simulink model "RobotDoSrodka10cmLimitZaokragloneNapSim"  (R2018a)
settings: Solver=ode45  StartTime=0.0  StopTime=tsym  RelTol=1e-6
values from neighbouring files (symbols this model uses):
  k1 = 10    [RobotDoSrodka10cmLimitZaokragloneNap.m]
  k2 = 100    [RobotDoSrodka10cmLimitZaokragloneNap.m]
  l = 0.0965    [RobotDoSrodka10cmLimitZaokragloneNap.m]
  R = 0.034    [RobotDoSrodka10cmLimitZaokragloneNap.m]
  wheelSpeedRadiansLimit = 8    [RobotDoSrodka10cmLimitZaokragloneNap.m]
undefined symbols (not defined in the file or in its folder): wd
settings Model: Creator=Papa Smerf  LastModifiedBy=Papa Smerf
settings DataIOCC: LimitDataPoints=on  SaveFormat=Array
settings OptimizationCC: BlockReduction=off  BooleanDataType=off  LifeSpan=inf
settings DebuggingCC: SaveWithParameterizedLinksMsg=none  UnderspecifiedInitializationDetection=Classic  MergeDetectMultiDrivingBlocksExec=none  SignalResolutionControl=TryResolveAllWithWarning  SFUnexpectedBacktrackingDiag=warning  SFNoUnconditionalDefaultTransitionDiag=warning  SFExecutionAtInitializationDiag=none
settings HardwareCC: ProdBitPerPointer=32  ProdBitPerSizeT=32  ProdBitPerPtrDiffT=32  ProdLargestAtomicFloat=None  ProdIntDivRoundTo=Undefined  ProdEndianess=Unspecified  ProdWordSize=32  ProdHWDeviceType=32-bit Generic  TargetUnknown=on
settings ModelReferenceCC: PropagateSignalLabelsOutOfModel=off
settings CodeAppCC: StateflowObjectComments=on
settings GRTTargetCC: TargetLangStandard=C89/C90 (ANSI)  GeneratePreprocessorConditionals=Disable all
settings ConfigComp: CovMetricSettings=dw  CovHtmlReporting=on  CovSaveCumulativeToWorkspaceVar=on  CovSaveSingleToWorkspaceVar=on  CovExternalEMLEnable=off  CovSFcnEnable=off

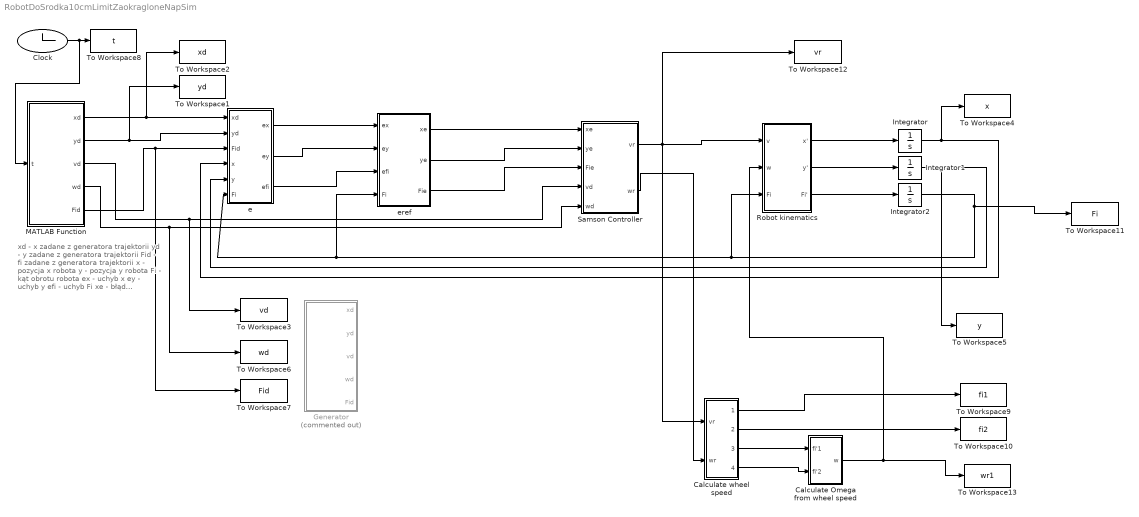
== system RobotDoSrodka10cmLimitZaokragloneNapSim ==
  note: xd - x zadane z generatora trajektorii
      | yd - y zadane z generatora trajektorii
      | Fid - fi zadane z generatora trajektorii
      | x - pozycja x robota
      | y - pozycja y robota
      | Fi - kąt obrotu robota
      | ex - uchyb x
      | ey - uchyb y
      | efi - uchyb Fi
      | xe - błąd referencyjny x
      | ye - błąd referencyjny y
      | Fie - błąd referencyjny Fi
      | vd - prędkość liniowa zadana
      | wd - prędkość kątowa zadana
      | vr - prędkość liniowa referencyjna
      | wr - prędkość kątowa referencyjna
      | v - prędkość liniowa zadana robota?
      | w - prędkość kątowa zadana robota?
      | x' - prędkość w osi x robota
      | y' - prędkość w osi y robota
      | Fi' - prędkość kątowa robota
  Calculate Omega from wheel speed : Subsystem
  Calculate wheel speed : Subsystem
  Clock : Clock
  Generator : Subsystem  Commented=on
  Integrator : Integrator
  Integrator1 : Integrator
  Integrator2 : Integrator
  MATLAB Function : MATLAB Function  TreatAsAtomicUnit=on
  Robot kinematics : Subsystem
  Samson Controller : Subsystem
  To Workspace1 : ToWorkspace  VariableName=yd  SampleTime=-1
  To Workspace10 : ToWorkspace  VariableName=fi2  SampleTime=0.01
  To Workspace11 : ToWorkspace  VariableName=Fi  SampleTime=0.01
  To Workspace12 : ToWorkspace  VariableName=vr  SampleTime=0.01
  To Workspace13 : ToWorkspace  VariableName=wr1  SampleTime=0.01
  To Workspace2 : ToWorkspace  VariableName=xd  SampleTime=-1
  To Workspace3 : ToWorkspace  VariableName=vd  SampleTime=-1
  To Workspace4 : ToWorkspace  VariableName=x  SampleTime=-1
  To Workspace5 : ToWorkspace  VariableName=y  SampleTime=-1
  To Workspace6 : ToWorkspace  VariableName=wd  SampleTime=-1
  To Workspace7 : ToWorkspace  VariableName=Fid  SampleTime=0.01
  To Workspace8 : ToWorkspace  VariableName=t  SampleTime=0.01
  To Workspace9 : ToWorkspace  VariableName=fi1  SampleTime=0.01
  e : Subsystem
  eref : Subsystem
  wires:
  e/1(ex) -> eref/1(ex)
  e/2(ey) -> eref/2(ey)
  e/3(efi) -> eref/3(efi)
  eref/1(xe) -> Samson Controller/1(xe)
  eref/2(ye) -> Samson Controller/2(ye)
  eref/3(Fie) -> Samson Controller/3(Fie)
  Robot kinematics/1(x') -> Integrator/1
  Robot kinematics/2(y') -> Integrator1/1
  Robot kinematics/3(Fi') -> Integrator2/1
  Integrator2/1 -> To Workspace11/1, Robot kinematics/3(Fi), e/6(Fi), eref/4(Fi)
  Integrator1/1 -> To Workspace5/1, e/5(y)
  Integrator/1 -> To Workspace4/1, e/4(x)
  MATLAB Function/1(xd) -> To Workspace2/1, e/1(xd)
  MATLAB Function/2(yd) -> To Workspace1/1, e/2(yd)
  MATLAB Function/5(Fid) -> To Workspace7/1, e/3(Fid)
  MATLAB Function/3(vd) -> To Workspace3/1, Samson Controller/4(vd)
  MATLAB Function/4(wd) -> To Workspace6/1, Samson Controller/5(wd)
  Clock/1 -> MATLAB Function/1(t), To Workspace8/1
  Calculate Omega from wheel speed/1(w) -> Robot kinematics/2(w), To Workspace13/1
  Calculate wheel speed/3(fi'1Rad) -> Calculate Omega from wheel speed/1(fi'1)
  Samson Controller/2(wr) -> Calculate wheel speed/2(wr)
  Calculate wheel speed/2(fi'2Obr) -> To Workspace10/1
  Calculate wheel speed/4(fi'2Rad) -> Calculate Omega from wheel speed/2(fi'2)
  Samson Controller/1(vr) -> Calculate wheel speed/1(vr), To Workspace12/1, Robot kinematics/1(v)
  Calculate wheel speed/1(fi'1Obr) -> To Workspace9/1

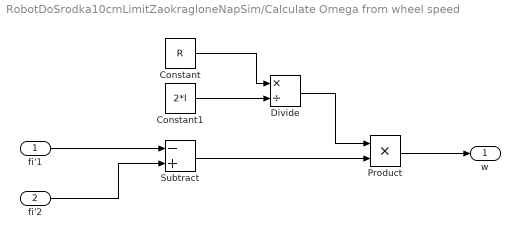
== system RobotDoSrodka10cmLimitZaokragloneNapSim/Calculate Omega from wheel speed ==
  fi'1 : Inport
  fi'2 : Inport  Port=2
  Constant : Constant  Value=R
  Constant1 : Constant  Value=2*l
  Divide : Product  Inputs=*/
  Product : Product
  Subtract : Sum  Inputs=-+
  w : Outport
  wires:
  Constant/1 -> Divide/1
  Product/1 -> w/1
  Subtract/1 -> Product/2
  Constant1/1 -> Divide/2
  fi'2/1 -> Subtract/2
  fi'1/1 -> Subtract/1
  Divide/1 -> Product/1

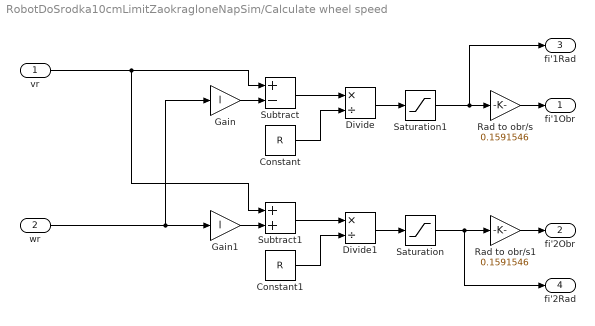
== system RobotDoSrodka10cmLimitZaokragloneNapSim/Calculate wheel speed ==
  vr : Inport
  wr : Inport  Port=2
  Constant : Constant  Value=R
  Constant1 : Constant  Value=R
  Divide : Product  Inputs=*/
  Divide1 : Product  Inputs=*/
  Gain : Gain  Gain=l
  Gain1 : Gain  Gain=l
  Rad to obr/s : Gain  Gain=0.1591546
  Rad to obr/s1 : Gain  Gain=0.1591546
  Saturation : Saturate  UpperLimit=wheelSpeedRadiansLimit  LowerLimit=-wheelSpeedRadiansLimit
  Saturation1 : Saturate  UpperLimit=wheelSpeedRadiansLimit  LowerLimit=-wheelSpeedRadiansLimit
  Subtract : Sum  Inputs=+-
  Subtract1 : Sum
  fi'1Obr : Outport
  fi'2Obr : Outport  Port=2
  fi'1Rad : Outport  Port=3
  fi'2Rad : Outport  Port=4
  wires:
  Rad to obr/s/1 -> fi'1Obr/1
  wr/1 -> Gain/1, Gain1/1
  Constant1/1 -> Divide1/2
  Subtract1/1 -> Divide1/1
  Gain/1 -> Subtract/2
  Constant/1 -> Divide/2
  Subtract/1 -> Divide/1
  Gain1/1 -> Subtract1/2
  Divide/1 -> Saturation1/1
  Divide1/1 -> Saturation/1
  Rad to obr/s1/1 -> fi'2Obr/1
  vr/1 -> Subtract1/1, Subtract/1
  Saturation/1 -> fi'2Rad/1, Rad to obr/s1/1
  Saturation1/1 -> fi'1Rad/1, Rad to obr/s/1

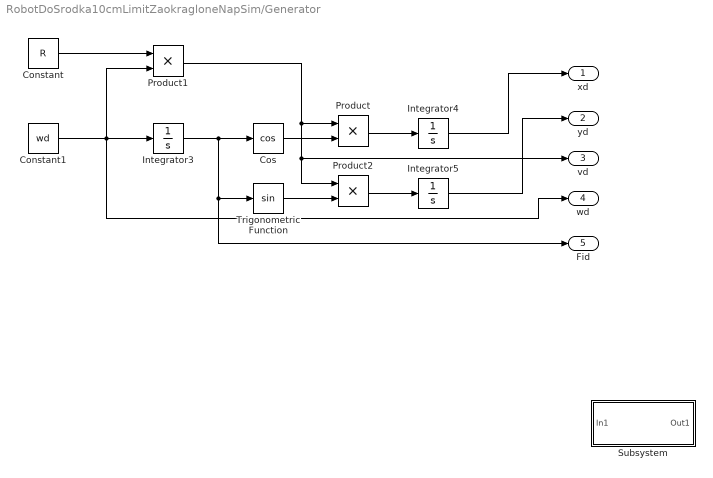
== system RobotDoSrodka10cmLimitZaokragloneNapSim/Generator ==
  Constant : Constant  Value=R
  Constant1 : Constant  Value=wd
  Cos : Trigonometry  Operator=cos
  Integrator3 : Integrator
  Integrator4 : Integrator
  Integrator5 : Integrator  InitialCondition=-R
  Product : Product
  Product1 : Product
  Product2 : Product
  Subsystem : Subsystem
  Trigonometric Function : Trigonometry
  xd : Outport
  yd : Outport  Port=2
  vd : Outport  Port=3
  wd : Outport  Port=4
  Fid : Outport  Port=5
  wires:
  Integrator5/1 -> yd/1
  Product1/1 -> vd/1, Product2/1, Product/1
  Constant/1 -> Product1/1
  Integrator3/1 -> Fid/1, Trigonometric Function/1, Cos/1
  Trigonometric Function/1 -> Product2/2
  Product/1 -> Integrator4/1
  Constant1/1 -> wd/1, Product1/2, Integrator3/1
  Cos/1 -> Product/2
  Integrator4/1 -> xd/1
  Product2/1 -> Integrator5/1

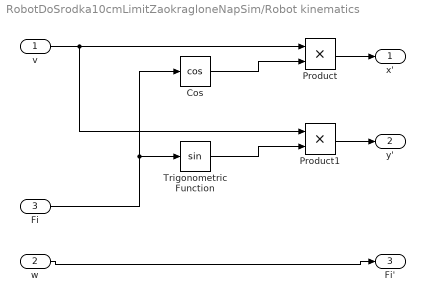
== system RobotDoSrodka10cmLimitZaokragloneNapSim/Robot kinematics ==
  v : Inport
  w : Inport  Port=2
  Fi : Inport  Port=3
  Cos : Trigonometry  Operator=cos
  Product : Product
  Product1 : Product
  Trigonometric Function : Trigonometry
  x' : Outport
  y' : Outport  Port=2
  Fi' : Outport  Port=3
  wires:
  w/1 -> Fi'/1
  Fi/1 -> Cos/1, Trigonometric Function/1
  Product1/1 -> y'/1
  v/1 -> Product1/1, Product/1
  Cos/1 -> Product/2
  Product/1 -> x'/1
  Trigonometric Function/1 -> Product1/2

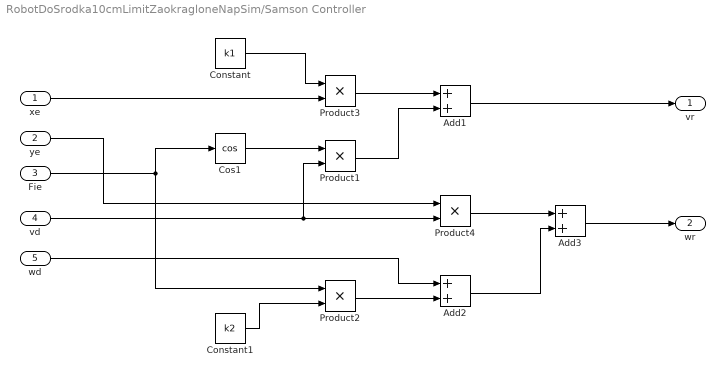
== system RobotDoSrodka10cmLimitZaokragloneNapSim/Samson Controller ==
  xe : Inport
  ye : Inport  Port=2
  Fie : Inport  Port=3
  vd : Inport  Port=4
  wd : Inport  Port=5
  Add1 : Sum
  Add2 : Sum
  Add3 : Sum
  Constant : Constant  Value=k1
  Constant1 : Constant  Value=k2
  Cos1 : Trigonometry  Operator=cos
  Product{1..4} (4 alike) : Product
  vr : Outport
  wr : Outport  Port=2
  wires:
  ye/1 -> Product4/1
  Fie/1 -> Product2/1, Cos1/1
  vd/1 -> Product4/2, Product1/2
  Add2/1 -> Add3/2
  Cos1/1 -> Product1/1
  xe/1 -> Product3/2
  Product3/1 -> Add1/1
  Product2/1 -> Add2/2
  Product1/1 -> Add1/2
  Add3/1 -> wr/1
  Add1/1 -> vr/1
  Constant/1 -> Product3/1
  Constant1/1 -> Product2/2
  wd/1 -> Add2/1
  Product4/1 -> Add3/1

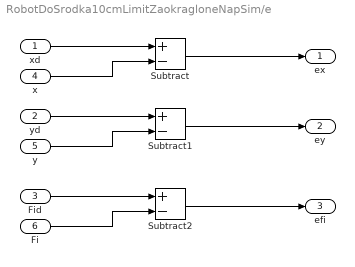
== system RobotDoSrodka10cmLimitZaokragloneNapSim/e ==
  xd : Inport
  yd : Inport  Port=2
  Fid : Inport  Port=3
  x : Inport  Port=4
  y : Inport  Port=5
  Fi : Inport  Port=6
  Subtract : Sum  Inputs=+-
  Subtract1 : Sum  Inputs=+-
  Subtract2 : Sum  Inputs=+-
  ex : Outport
  ey : Outport  Port=2
  efi : Outport  Port=3
  wires:
  Subtract/1 -> ex/1
  xd/1 -> Subtract/1
  Fi/1 -> Subtract2/2
  x/1 -> Subtract/2
  Subtract2/1 -> efi/1
  Fid/1 -> Subtract2/1
  Subtract1/1 -> ey/1
  yd/1 -> Subtract1/1
  y/1 -> Subtract1/2

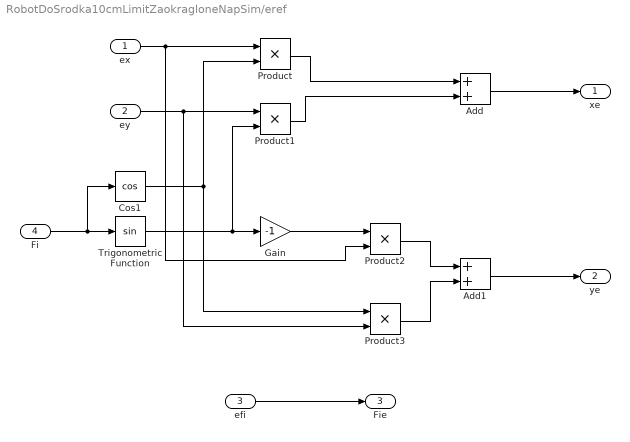
== system RobotDoSrodka10cmLimitZaokragloneNapSim/eref ==
  ex : Inport
  ey : Inport  Port=2
  efi : Inport  Port=3
  Fi : Inport  Port=4
  Add : Sum
  Add1 : Sum
  Cos1 : Trigonometry  Operator=cos
  Gain : Gain  Gain=-1
  Product{,1..3} (4 alike) : Product
  Trigonometric Function : Trigonometry
  xe : Outport
  ye : Outport  Port=2
  Fie : Outport  Port=3
  wires:
  Cos1/1 -> Product3/1, Product/2
  Product1/1 -> Add/2
  ey/1 -> Product3/2, Product1/1
  Add/1 -> xe/1
  Trigonometric Function/1 -> Product1/2, Gain/1
  Fi/1 -> Cos1/1, Trigonometric Function/1
  Product3/1 -> Add1/2
  Product/1 -> Add/1
  Add1/1 -> ye/1
  ex/1 -> Product2/2, Product/1
  Gain/1 -> Product2/1
  efi/1 -> Fie/1
  Product2/1 -> Add1/1

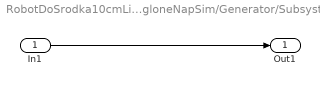
== system RobotDoSrodka10cmLimitZaokragloneNapSim/Generator/Subsystem ==
  In1 : Inport
  Out1 : Outport
  wires:
  In1/1 -> Out1/1

== matlab function RobotDoSrodka10cmLimitZaokragloneNapSim/MATLAB Function ==
  data: t input; xd output; yd output; vd output; wd output; Fid output
function [xd, yd, vd, wd, Fid] = fcn(t)

xd=0;
yd=0;
Fid=0;
vd=0.1;
wd=0;
speed = pi/2*1/2;
l = 0.0965;
if t<=9
    xd=vd*t;
    yd=0;
    Fid=0;
elseif ((t > 9) && (t <= 11))
    fi = speed * (t-9) - pi/2;
    xd=0.1*cos(fi) + 0.9;
    yd=0.1+ 0.1*sin(fi);
    Fid=fi+pi/2;
    wd = pi/2/2;
    vd = wd * l;
elseif ((t>11) && (t<=19))
    xd=1;
    yd=0.1+ (vd*t-1.1);
    Fid=pi/2;
    vd=0.1;
    wd=0;
elseif ((t>19) && (t<=21))
    fi = speed * (t-19);
    xd=0.1*cos(fi) + 1 - 0.1;
    yd=0.1+ 0.1*sin(fi) + 0.9 - 0.1;
    Fid=fi+pi/2;
    wd = pi/2/2;
    vd = wd * l;
elseif ((t>21) && (t<=29))
    xd=1-(vd*t-2);
    yd=1;
    Fid=pi;
    vd=0.1;
    wd=0;
elseif ((t>29) && (t<=31))
    fi = speed * (t-29) + pi/2;
    xd=0.1*cos(fi) + 0.1;
    yd=0.1+ 0.1*sin(fi) + 0.9 - 0.1;
    Fid=fi+pi/2;
    wd = pi/2/2;
    vd = wd * l;
elseif ((t>31) && (t<=37))
    xd=0;
    yd=0.9-(vd*t-3.1);
    Fid=3/2*pi;
    vd=0.1;
    wd=0;
elseif ((t>37) && (t<=39))
    fi = speed * (t-37) + pi;
    xd=0.1*cos(fi) + 0.1;
    yd=0.1+ 0.1*sin(fi) + 0.3 - 0.1;
    Fid=fi+pi/2;
    wd = pi/2/2;
    vd = wd * l;
elseif ((t>39) && (t<=45))
    xd=vd*t-3.9 + 0.1;
    yd=0.2;
    Fid=0 + 2*pi; 
    vd=0.1;
    wd=0;
elseif ((t > 45) && (t <= 47))
    fi = speed * (t-45) - pi/2+ 2*pi;
    xd=0.1*cos(fi) + 0.7;
    yd=0.1+ 0.1*sin(fi)+0.2;
    Fid=fi+pi/2;
    wd = pi/2/2;
    vd = wd * l;
elseif ((t>47) && (t<=51))
    xd= 0.8;
    yd= 0.3 +(vd*t-4.7);
    Fid=pi/2+ 2*pi;
    vd=0.1;
    wd=0;
elseif ((t>51) && (t<=53))
    fi = speed * (t-51)+ 2*pi;
    xd=0.1*cos(fi) + 0.8 - 0.1;
    yd=0.1+ 0.1*sin(fi) + 0.7 - 0.1;
    Fid=fi+pi/2;
    wd = pi/2/2;
    vd = wd * l;
elseif ((t>53) && (t<=57))
    xd=0.7-(vd*t-5.3);
    yd=0.8;
    Fid=pi+ 2*pi;
    vd=0.1;
    wd=0;
elseif ((t>57) && (t<=59))
    fi = speed * (t-57) + pi/2+ 2*pi;
    xd=0.1*cos(fi) + 0.1 + 0.2;
    yd=0.1+ 0.1*sin(fi) + 0.7 - 0.1;
    Fid=fi+pi/2;
    wd = pi/2/2;
    vd = wd * l;
elseif ((t>59) && (t<=61))
    xd=0.2;
    yd=0.7-(vd*t-5.9);
    Fid=3/2*pi+ 2*pi;
    vd=0.1;
    wd=0;
elseif ((t>61) && (t<=63))
    fi = speed * (t-61) + pi + 2*pi;
    xd=0.1*cos(fi) + 0.3;
    yd=0.1+ 0.1*sin(fi) + 0.5 - 0.1;
    Fid=fi+pi/2;
    wd = pi/2/2;
    vd = wd * l;
elseif ((t>63) && (t<=65))
    xd=0.3 + vd*t-6.3;
    yd=0.4;
    Fid=0 + 4*pi;  
    vd=0.1;
    wd=0;
elseif ((t > 65) && (t <= 69))
    fi = speed * (t-65) - pi/2+ 4*pi;
    xd=0.1*cos(fi) + 0.5;
    yd=0.1+ 0.1*sin(fi)+0.4;
    Fid=fi+pi/2;
    wd = pi/2/2;
    vd = wd * l;
elseif ((t>69) && (t<=70))
    xd= 0.5 -(vd*t-6.9);
    yd= 0.6;
    Fid=pi+ 4*pi;
    vd=0.1;
    wd=0;
elseif (t>70)
    xd=0.4;
    yd=0.6;
    Fid=pi+ 4*pi;
    vd=0;
    wd=0;
end
